simulink model "lht_1920_1080"  (R2020a)
settings: Solver=FixedStepDiscrete  StartTime=0.0  StopTime=inf  RelTol=1e-3
InitFcn:
  | setup_parallel_hough_transform;
StopFcn:
  | stop_parallel_hough_accumulator;
values from neighbouring files (symbols this model uses):
  bitsRho = ceil(log2(maxRho*2))    [setup_parallel_hough_transform.m]
  height = 1080    [setup_parallel_hough_transform.m]
  inarray = uint8(fi(edge, 0, 1, 0))    [setup_parallel_hough_transform.m]
  width = 1920    [setup_parallel_hough_transform.m]
undefined symbols (not defined in the file or in its folder): nTheta
libraries: hdlsllib x20, simulink x17, dspsrcs4 x1
(part 2 of 2)

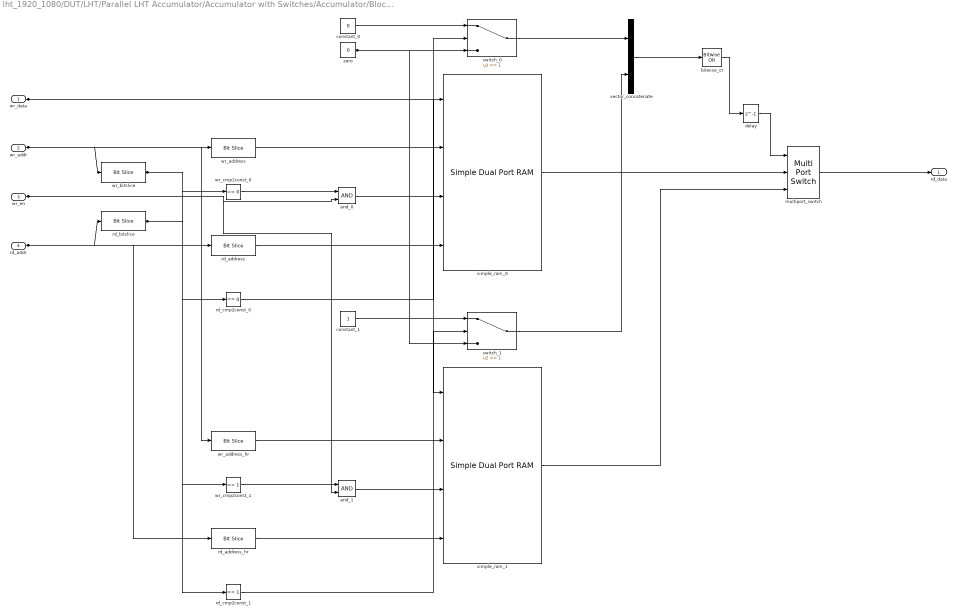
== system lht_1920_1080/DUT/LHT/Parallel LHT Accumulator/Accumulator with Switches/Accumulator/Block RAM/Simple Dual Port RAM Generator ==
  wr_data : Inport
  wr_addr : Inport  Port=2
  wr_en : Inport  Port=3
  rd_addr : Inport  Port=4
  and_0 : Logic  AllPortsSameDT=off  OutDataTypeStr=boolean
  and_1 : Logic  AllPortsSameDT=off  OutDataTypeStr=boolean
  bitwise_or : simulink/Logic and Bit Operations/Bitwise Operator  logicop=OR  UseBitMask=off  BitMask=bin2dec('11011001')  BitMaskRealWorld=Stored Integer
  constant_0 : Constant  Value=0  OutDataTypeStr=fixdt(0, 2, 0)  SampleTime=-1
  constant_1 : Constant  OutDataTypeStr=fixdt(0, 2, 0)  SampleTime=-1
  delay : Delay  DelayLength=1
  multiport_switch : MultiPortSwitch  DataPortOrder=Zero-based contiguous  Inputs=2  zeroidx=on
  rd_address : hdlsllib/Logic and Bit Operations/Bit Slice  lidx=10  ridx=0
      settings: SourceProductBaseCode=SL
  rd_address_hr : hdlsllib/Logic and Bit Operations/Bit Slice  lidx=9  ridx=0
      settings: SourceProductBaseCode=SL
  rd_bitslice : hdlsllib/Logic and Bit Operations/Bit Slice  lidx=11  ridx=11
      settings: SourceProductBaseCode=SL
  rd_cmp2const_0 : simulink/Logic and Bit Operations/Compare To Constant  relop===  const=0  OutDataTypeStr=boolean
  rd_cmp2const_1 : simulink/Logic and Bit Operations/Compare To Constant  relop===  const=1  OutDataTypeStr=boolean
  simple_ram_0 : hdlsllib/HDL RAMs/Simple Dual Port RAM  ram_size=11
      settings: SourceProductBaseCode=SL
  simple_ram_1 : hdlsllib/HDL RAMs/Simple Dual Port RAM  ram_size=10
      settings: SourceProductBaseCode=SL
  switch_0 : Switch  Threshold=1
  switch_1 : Switch  Threshold=1
  vector_concatenate : Concatenate
  wr_address : hdlsllib/Logic and Bit Operations/Bit Slice  lidx=10  ridx=0
      settings: SourceProductBaseCode=SL
  wr_address_hr : hdlsllib/Logic and Bit Operations/Bit Slice  lidx=9  ridx=0
      settings: SourceProductBaseCode=SL
  wr_bitslice : hdlsllib/Logic and Bit Operations/Bit Slice  lidx=11  ridx=11
      settings: SourceProductBaseCode=SL
  wr_cmp2const_0 : simulink/Logic and Bit Operations/Compare To Constant  relop===  const=0  OutDataTypeStr=boolean
  wr_cmp2const_1 : simulink/Logic and Bit Operations/Compare To Constant  relop===  const=1  OutDataTypeStr=boolean
  zero : Constant  Value=0  OutDataTypeStr=fixdt(0, 2, 0)  SampleTime=-1
  rd_data : Outport
  wires:
  wr_data/1 -> simple_ram_0/1, simple_ram_1/1
  wr_address/1 -> simple_ram_0/2
  rd_address/1 -> simple_ram_0/4
  constant_0/1 -> switch_0/1
  zero/1 -> switch_0/3, switch_1/3
  switch_0/1 -> vector_concatenate/1
  simple_ram_0/1 -> multiport_switch/2
  wr_bitslice/1 -> wr_cmp2const_0/1, wr_cmp2const_1/1
  rd_bitslice/1 -> rd_cmp2const_0/1, rd_cmp2const_1/1
  wr_en/1 -> and_0/2, and_1/2
  and_0/1 -> simple_ram_0/3
  wr_cmp2const_0/1 -> and_0/1
  rd_cmp2const_0/1 -> switch_0/2
  constant_1/1 -> switch_1/1
  switch_1/1 -> vector_concatenate/2
  simple_ram_1/1 -> multiport_switch/3
  and_1/1 -> simple_ram_1/3
  wr_cmp2const_1/1 -> and_1/1
  rd_cmp2const_1/1 -> switch_1/2
  rd_addr/1 -> rd_bitslice/1, rd_address/1, rd_address_hr/1
  wr_addr/1 -> wr_bitslice/1, wr_address/1, wr_address_hr/1
  vector_concatenate/1 -> bitwise_or/1
  bitwise_or/1 -> delay/1
  delay/1 -> multiport_switch/1
  multiport_switch/1 -> rd_data/1
  wr_address_hr/1 -> simple_ram_1/2
  rd_address_hr/1 -> simple_ram_1/4

== matlab function lht_1920_1080/DUT/LHT/Parallel LHT Accumulator/Accumulator Controller ==
  data: sof input; mode output; eof input; read output; clear output; index output; ntheta input; nrho input; valid output; debug_state output
function [mode, read, clear, index, valid, debug_state] = fcn(sof, eof, ntheta, nrho)

IDLE = fi(0, 0, 2, 0);
VOTE = fi(1, 0, 2, 0);
READ = fi(2, 0, 2, 0);
CLEAR = fi(3, 0, 2, 0);

persistent current_state;
persistent rho_counter;
persistent theta_counter;

if isempty(current_state)
    current_state = IDLE;
end

if isempty(rho_counter)
    rho_counter = fi(0, 0, 16, 0);
end

if isempty(theta_counter)
    theta_counter = fi(0, 0, 16, 0);
end

switch current_state
    case IDLE
        rho_counter = fi(0, 0, 16, 0);
        theta_counter = fi(0, 0, 16, 0);
        
        clear = false;
        read = rho_counter;
        index = theta_counter;
        valid = false;
        debug_state = current_state;
        
        if sof
            mode = true;
            current_state = VOTE;
        else
            mode = false;
            current_state = IDLE;
        end
        
    case VOTE
        rho_counter = fi(0, 0, 16, 0);
        theta_counter = fi(0, 0, 16, 0);
        
        mode = true;
        clear = false;
        valid = false;
        debug_state = current_state;
        
        read = rho_counter;
        index = theta_counter;
        
        if eof
            current_state = READ;
        else
            current_state = VOTE;
        end
        
    case READ
        mode = false;
        clear = false;
        read = rho_counter;
        index = theta_counter;
        valid = true;
        debug_state = current_state;
        
        if theta_counter >= ntheta && rho_counter >= nrho
            rho_counter = fi(0, 0, 16, 0);
            theta_counter = fi(0, 0, 16, 0);
            current_state = CLEAR;
        elseif rho_counter >= nrho
            theta_counter = fi(theta_counter + 1, 0, 16, 0);
            rho_counter = fi(0, 0, 16, 0);
            current_state = READ;
        else
            rho_counter = fi(rho_counter + 1, 0, 16, 0);
            current_state = READ;
        end
        
    case CLEAR
        mode = false;
        clear = true;
        valid = false;
        
        read = rho_counter;
        index = theta_counter;
        debug_state = current_state;
        
        if rho_counter >= nrho
            rho_counter = fi(0, 0, 16, 0);
            theta_counter = fi(0, 0, 16, 0);
            current_state = IDLE;
        else
            rho_counter = fi(rho_counter + 1, 0, 16, 0);
            theta_counter = fi(0, 0, 16, 0);
            current_state = CLEAR;
        end
        
    otherwise
        rho_counter = fi(0, 0, 16, 0);
        theta_counter = fi(0, 0, 16, 0);
        
        mode = false;
        clear = false;
        valid = false;
        debug_state = current_state;
        
        read = rho_counter;
        index = theta_counter;
        
        current_state = IDLE;
        
end
